simulink model "schema_di_controllo_progetto"  (R2023b)
settings: Solver=VariableStepAuto  StartTime=0.0  StopTime=1  RelTol=1e-3
values from neighbouring files (symbols this model uses):
  C_eq = double(subs(C, symbols, values))    [progetto_B3_AK.m]
  u_eq = 85/9*pi    (= 29.6705972839)    [progetto_B3_AK.m]
  w = 3    [progetto_B3_AK.m]
  x_eq = [17/36*pi; 0]    [progetto_B3_AK.m]
libraries: cstblocks x1
settings Model: SimulationMode=rapid-accelerator  Creator=guidocarnevale  LastModifiedBy=pierr

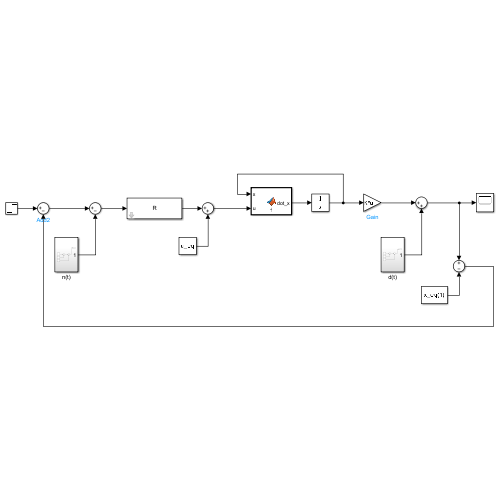
[thumbnail: Simulink's stored preview of the top-level diagram]
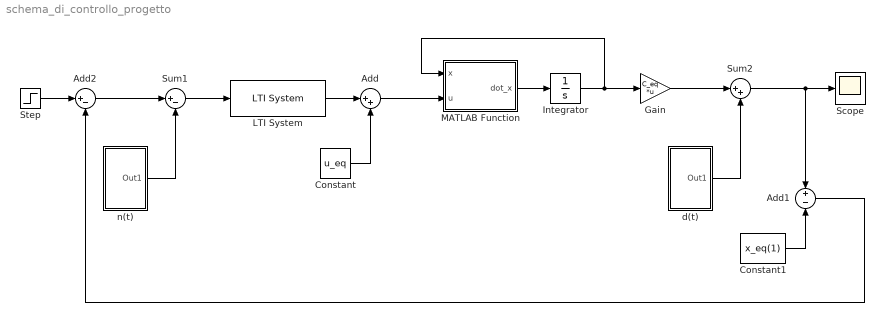
== system schema_di_controllo_progetto ==
  Add : Sum  Inputs=|++
  Add1 : Sum  Inputs=+|-
  Add2 : Sum  Inputs=|+-
  Constant : Constant  Value=u_eq
  Constant1 : Constant  Value=x_eq(1)
  Gain : Gain  Gain=C_eq  Multiplication=Matrix(K*u)
  Integrator : Integrator  InitialCondition=[x_eq(1) + 100;x_eq(2) + 100]
  LTI System : cstblocks/LTI System  sys=R  IC=[]  PadeOrder=0
  MATLAB Function : MATLAB Function  TreatAsAtomicUnit=on
  Scope : Scope
  Step : Step  Time=0  After=w  SampleTime=0
  Sum1 : Sum  Inputs=|+-
  Sum2 : Sum  Inputs=|++
  d(t) : Subsystem
  n(t) : Subsystem
  wires:
  MATLAB Function/1(dot_x) -> Integrator/1
  Integrator/1 -> MATLAB Function/1(x), Gain/1
  Constant/1 -> Add/2
  LTI System/1 -> Add/1
  Add/1 -> MATLAB Function/2(u)
  Constant1/1 -> Add1/2
  Add1/1 -> Add2/2
  Step/1 -> Add2/1
  Sum1/1 -> LTI System/1
  Add2/1 -> Sum1/1
  n(t)/1(Out1) -> Sum1/2
  Gain/1 -> Sum2/1
  d(t)/1(Out1) -> Sum2/2
  Sum2/1 -> Scope/1, Add1/1

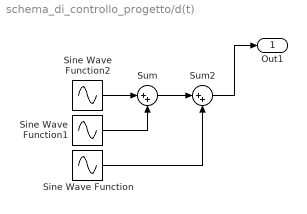
== system schema_di_controllo_progetto/d(t) ==
  Sine Wave Function : Sin  Amplitude=3  Frequency=0.01  SampleTime=0
  Sine Wave Function1 : Sin  Amplitude=3  Frequency=0.02  SampleTime=0
  Sine Wave Function2 : Sin  Amplitude=3  Frequency=0.03  SampleTime=0
  Sum : Sum  Inputs=|++
  Sum2 : Sum  Inputs=|++
  Out1 : Outport
  wires:
  Sine Wave Function2/1 -> Sum/1
  Sum/1 -> Sum2/1
  Sine Wave Function/1 -> Sum2/2
  Sum2/1 -> Out1/1
  Sine Wave Function1/1 -> Sum/2

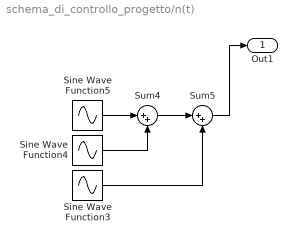
== system schema_di_controllo_progetto/n(t) ==
  Sine Wave Function3 : Sin  Amplitude=3  Frequency=3e5  SampleTime=0
  Sine Wave Function4 : Sin  Amplitude=3  Frequency=2e5  SampleTime=0
  Sine Wave Function5 : Sin  Amplitude=3  Frequency=1e5  SampleTime=0
  Sum4 : Sum  Inputs=|++
  Sum5 : Sum  Inputs=|++
  Out1 : Outport
  wires:
  Sine Wave Function3/1 -> Sum5/2
  Sine Wave Function5/1 -> Sum4/1
  Sum5/1 -> Out1/1
  Sine Wave Function4/1 -> Sum4/2
  Sum4/1 -> Sum5/1

== matlab function schema_di_controllo_progetto/MATLAB Function ==
  data: x input; u input; dot_x output
function dot_x = f(x,u)

%%%%%%%%%%%%%%%%%%%%%%%%%%%%%%%%%
% system parametres
%%%%%%%%%%%%%%%%%%%%%%%%%%%%%%%%%
J_0   = 2;
J    = [0.5 0.01 0.01 0.08];
phi  = [-1 2 1.5 -2];
beta  = 0.2;
k    = 20;

%%%%%%%%%%%%%%%%%%%%%%%%%%%
% J(x)
%%%%%%%%%%%%%%%%%%%%%%%%%%%
l           = 4;

J_x         = J_0;
for i = 1:l
    J_x     = J_x + J(i)*cos(i*x(1)+phi(i));
end


dot_x = zeros(2,1);

dot_x(1) = x(2);

dot_x(2) =  1/J_x * (u - beta*x(2) - k*x(1));
